simulink model "c00019M_harness"  (R2018a)
settings: Solver=ode3  StartTime=0.0  StopTime=10.0  RelTol=1e-3  EnableMultiTasking=on
undefined symbols (not defined in the file): b, DiscIntNeverNeededParam, J, K, L, PosMinimaW4, R, sigbuilder_block
(part 13 of 43)

== system c00019M_harness/M094/Cyber ==
  note: Sensors
  note: Inputs For Window1
  note: Inputs for Window 2
  note: Inputs for window 3
  note: Inputs for window 4
  note: Users
  note: Users
  note: Sensors
  note: Users
  note: Sensors
  note: Users
  note: Sensors
  note: USERS
      | ---------------------------------
      | 0: None
      | 1: Ventana Arriba
      | 2: Ventana hasta arriba
      | 3: Ventana abajo
      | 4: Ventana hasta abajo
  note: 1: SUBE
      | 0: PARADO
      | -1 BAJA
  note: D = Driver (W1)
      | P1 = Passenger 1 (W2)
      | P2 = Passenger 2 (W3)
      | P3 = Passenger 3 (W4)
      | O = Obstacle
      | C = Control
      | Pri = Prioritizer
      | LD = LockDriver
      | PosW = PositionWindow
      | WL = WindowLogic
      | OW = ObstacleWindow
      | CWXC = ControlWindowXCentralized
      | S = Sensor
      | L = Lock
      | WPos = WindowPosition
      | M = Memory
      | InW = InputWindow
      | WIn = WindowInput
  PosW1 : Inport
  PosW2 : Inport  Port=2
  PosW4 : Inport  Port=3
  DW1 : Inport  Port=4
  P1W2 : Inport  Port=5
  P3W4 : Inport  Port=6
  OW1 : Inport  Port=7
  OW2 : Inport  Port=8
  OW4 : Inport  Port=9
  LD : Inport  Port=10
  CW1C : Inport  Port=11
  CW2C : Inport  Port=12
  CW4C : Inport  Port=13
  Pri : Subsystem
  Pri3 : Subsystem
  Pri4 : Subsystem
  WL : Subsystem
  WL1 : Subsystem
  WL3 : Subsystem
  W1 : Outport
  W2 : Outport  Port=2
  W4 : Outport  Port=3
  wires:
  CW4C/1 -> Pri4/2(CW4C)
  CW2C/1 -> Pri/2(CW2C)
  CW1C/1 -> Pri3/2(CW1C)
  Pri3/1(User) -> WL/2(User)
  WL3/1(WindowLogicOutput) -> W4/1
  Pri4/1(User) -> WL3/2(User)
  OW4/1 -> WL3/3(OW)
  PosW4/1 -> WL3/1(WPos)
  P3W4/1 -> Pri4/1(P)
  WL1/1(WindowLogicOutput) -> W2/1
  OW2/1 -> WL1/3(OW)
  PosW2/1 -> WL1/1(WPos)
  P1W2/1 -> Pri/1(P)
  Pri/1(User) -> WL1/2(User)
  WL/1(WindowLogicOutput) -> W1/1
  DW1/1 -> Pri3/1(D)
  OW1/1 -> WL/3(OW)
  PosW1/1 -> WL/1(WPos)
  LD/1 -> WL3/4(L)

== system c00019M_harness/M094/Physical ==
  InW1 : Inport
  InW2 : Inport  Port=2
  InW4 : Inport  Port=3
  W : Subsystem
  W5 : Subsystem
  W7 : Subsystem
  W1 : Outport
  W2 : Outport  Port=2
  W4 : Outport  Port=3
  wires:
  W7/1(WPos) -> W4/1
  W5/1(WPos) -> W2/1
  W/1(WPos) -> W1/1
  InW4/1 -> W7/1(WIn)
  InW2/1 -> W5/1(WIn)
  InW1/1 -> W/1(WIn)

== system c00019M_harness/M094/S1 ==
  PhyMeasure : Inport
  SensorOut : Outport
  wires:
  PhyMeasure/1 -> SensorOut/1

== system c00019M_harness/M094/S2 ==
  PhyMeasure : Inport
  SensorOut : Outport
  wires:
  PhyMeasure/1 -> SensorOut/1

== system c00019M_harness/M094/S4 ==
  PhyMeasure : Inport
  SensorOut : Outport
  wires:
  PhyMeasure/1 -> SensorOut/1

== system c00019M_harness/M095/Cyber ==
  note: Sensors
  note: Inputs For Window1
  note: Inputs for Window 2
  note: Inputs for window 3
  note: Inputs for window 4
  note: Users
  note: Users
  note: Sensors
  note: Users
  note: Sensors
  note: Users
  note: Sensors
  note: USERS
      | ---------------------------------
      | 0: None
      | 1: Ventana Arriba
      | 2: Ventana hasta arriba
      | 3: Ventana abajo
      | 4: Ventana hasta abajo
  note: 1: SUBE
      | 0: PARADO
      | -1 BAJA
  note: D = Driver (W1)
      | P1 = Passenger 1 (W2)
      | P2 = Passenger 2 (W3)
      | P3 = Passenger 3 (W4)
      | O = Obstacle
      | C = Control
      | Pri = Prioritizer
      | LD = LockDriver
      | PosW = PositionWindow
      | WL = WindowLogic
      | OW = ObstacleWindow
      | CWXC = ControlWindowXCentralized
      | S = Sensor
      | L = Lock
      | WPos = WindowPosition
      | M = Memory
      | InW = InputWindow
      | WIn = WindowInput
  PosW1 : Inport
  PosW2 : Inport  Port=2
  PosW4 : Inport  Port=3
  DW1 : Inport  Port=4
  P1W2 : Inport  Port=5
  P3W4 : Inport  Port=6
  OW1 : Inport  Port=7
  OW2 : Inport  Port=8
  OW4 : Inport  Port=9
  LD : Inport  Port=10
  CW1C : Inport  Port=11
  CW2C : Inport  Port=12
  CW4C : Inport  Port=13
  Pri : Subsystem
  Pri3 : Subsystem
  Pri4 : Subsystem
  WL : Subsystem
  WL1 : Subsystem
  WL3 : Subsystem
  W1 : Outport
  W2 : Outport  Port=2
  W4 : Outport  Port=3
  wires:
  CW4C/1 -> Pri4/2(CW4C)
  CW2C/1 -> Pri/2(CW2C)
  CW1C/1 -> Pri3/2(CW1C)
  Pri3/1(User) -> WL/2(User)
  WL3/1(WindowLogicOutput) -> W4/1
  Pri4/1(User) -> WL3/2(User)
  OW4/1 -> WL3/3(OW)
  PosW4/1 -> WL3/1(WPos)
  P3W4/1 -> Pri4/1(P)
  WL1/1(WindowLogicOutput) -> W2/1
  OW2/1 -> WL1/3(OW)
  PosW2/1 -> WL1/1(WPos)
  P1W2/1 -> Pri/1(P)
  Pri/1(User) -> WL1/2(User)
  WL/1(WindowLogicOutput) -> W1/1
  DW1/1 -> Pri3/1(D)
  OW1/1 -> WL/3(OW)
  PosW1/1 -> WL/1(WPos)
  LD/1 -> WL3/4(L)

== system c00019M_harness/M095/Physical ==
  InW1 : Inport
  InW2 : Inport  Port=2
  InW4 : Inport  Port=3
  W : Subsystem
  W5 : Subsystem
  W7 : Subsystem
  W1 : Outport
  W2 : Outport  Port=2
  W4 : Outport  Port=3
  wires:
  W7/1(WPos) -> W4/1
  W5/1(WPos) -> W2/1
  W/1(WPos) -> W1/1
  InW4/1 -> W7/1(WIn)
  InW2/1 -> W5/1(WIn)
  InW1/1 -> W/1(WIn)

== system c00019M_harness/M095/S1 ==
  PhyMeasure : Inport
  SensorOut : Outport
  wires:
  PhyMeasure/1 -> SensorOut/1

== system c00019M_harness/M095/S2 ==
  PhyMeasure : Inport
  SensorOut : Outport
  wires:
  PhyMeasure/1 -> SensorOut/1

== system c00019M_harness/M095/S4 ==
  PhyMeasure : Inport
  SensorOut : Outport
  wires:
  PhyMeasure/1 -> SensorOut/1

== system c00019M_harness/M096/Cyber ==
  note: Sensors
  note: Inputs For Window1
  note: Inputs for Window 2
  note: Inputs for window 3
  note: Inputs for window 4
  note: Users
  note: Users
  note: Sensors
  note: Users
  note: Sensors
  note: Users
  note: Sensors
  note: USERS
      | ---------------------------------
      | 0: None
      | 1: Ventana Arriba
      | 2: Ventana hasta arriba
      | 3: Ventana abajo
      | 4: Ventana hasta abajo
  note: 1: SUBE
      | 0: PARADO
      | -1 BAJA
  note: D = Driver (W1)
      | P1 = Passenger 1 (W2)
      | P2 = Passenger 2 (W3)
      | P3 = Passenger 3 (W4)
      | O = Obstacle
      | C = Control
      | Pri = Prioritizer
      | LD = LockDriver
      | PosW = PositionWindow
      | WL = WindowLogic
      | OW = ObstacleWindow
      | CWXC = ControlWindowXCentralized
      | S = Sensor
      | L = Lock
      | WPos = WindowPosition
      | M = Memory
      | InW = InputWindow
      | WIn = WindowInput
  PosW1 : Inport
  PosW2 : Inport  Port=2
  PosW4 : Inport  Port=3
  DW1 : Inport  Port=4
  P1W2 : Inport  Port=5
  P3W4 : Inport  Port=6
  OW1 : Inport  Port=7
  OW2 : Inport  Port=8
  OW4 : Inport  Port=9
  LD : Inport  Port=10
  CW1C : Inport  Port=11
  CW2C : Inport  Port=12
  CW4C : Inport  Port=13
  Pri : Subsystem
  Pri3 : Subsystem
  Pri4 : Subsystem
  WL : Subsystem
  WL1 : Subsystem
  WL3 : Subsystem
  W1 : Outport
  W2 : Outport  Port=2
  W4 : Outport  Port=3
  wires:
  CW4C/1 -> Pri4/2(CW4C)
  CW2C/1 -> Pri/2(CW2C)
  CW1C/1 -> Pri3/2(CW1C)
  Pri3/1(User) -> WL/2(User)
  WL3/1(WindowLogicOutput) -> W4/1
  Pri4/1(User) -> WL3/2(User)
  OW4/1 -> WL3/3(OW)
  PosW4/1 -> WL3/1(WPos)
  P3W4/1 -> Pri4/1(P)
  WL1/1(WindowLogicOutput) -> W2/1
  OW2/1 -> WL1/3(OW)
  PosW2/1 -> WL1/1(WPos)
  P1W2/1 -> Pri/1(P)
  Pri/1(User) -> WL1/2(User)
  WL/1(WindowLogicOutput) -> W1/1
  DW1/1 -> Pri3/1(D)
  OW1/1 -> WL/3(OW)
  PosW1/1 -> WL/1(WPos)
  LD/1 -> WL3/4(L)

== system c00019M_harness/M096/Physical ==
  InW1 : Inport
  InW2 : Inport  Port=2
  InW4 : Inport  Port=3
  W : Subsystem
  W5 : Subsystem
  W7 : Subsystem
  W1 : Outport
  W2 : Outport  Port=2
  W4 : Outport  Port=3
  wires:
  W7/1(WPos) -> W4/1
  W5/1(WPos) -> W2/1
  W/1(WPos) -> W1/1
  InW4/1 -> W7/1(WIn)
  InW2/1 -> W5/1(WIn)
  InW1/1 -> W/1(WIn)

== system c00019M_harness/M096/S1 ==
  PhyMeasure : Inport
  SensorOut : Outport
  wires:
  PhyMeasure/1 -> SensorOut/1

== system c00019M_harness/M096/S2 ==
  PhyMeasure : Inport
  SensorOut : Outport
  wires:
  PhyMeasure/1 -> SensorOut/1

== system c00019M_harness/M096/S4 ==
  PhyMeasure : Inport
  SensorOut : Outport
  wires:
  PhyMeasure/1 -> SensorOut/1

== system c00019M_harness/M098/Cyber ==
  note: Sensors
  note: Inputs For Window1
  note: Inputs for Window 2
  note: Inputs for window 3
  note: Inputs for window 4
  note: Users
  note: Users
  note: Sensors
  note: Users
  note: Sensors
  note: Users
  note: Sensors
  note: USERS
      | ---------------------------------
      | 0: None
      | 1: Ventana Arriba
      | 2: Ventana hasta arriba
      | 3: Ventana abajo
      | 4: Ventana hasta abajo
  note: 1: SUBE
      | 0: PARADO
      | -1 BAJA
  note: D = Driver (W1)
      | P1 = Passenger 1 (W2)
      | P2 = Passenger 2 (W3)
      | P3 = Passenger 3 (W4)
      | O = Obstacle
      | C = Control
      | Pri = Prioritizer
      | LD = LockDriver
      | PosW = PositionWindow
      | WL = WindowLogic
      | OW = ObstacleWindow
      | CWXC = ControlWindowXCentralized
      | S = Sensor
      | L = Lock
      | WPos = WindowPosition
      | M = Memory
      | InW = InputWindow
      | WIn = WindowInput
  PosW1 : Inport
  PosW2 : Inport  Port=2
  PosW4 : Inport  Port=3
  DW1 : Inport  Port=4
  P1W2 : Inport  Port=5
  P3W4 : Inport  Port=6
  OW1 : Inport  Port=7
  OW2 : Inport  Port=8
  OW4 : Inport  Port=9
  LD : Inport  Port=10
  CW1C : Inport  Port=11
  CW2C : Inport  Port=12
  CW4C : Inport  Port=13
  Pri : Subsystem
  Pri3 : Subsystem
  Pri4 : Subsystem
  WL : Subsystem
  WL1 : Subsystem
  WL3 : Subsystem
  W1 : Outport
  W2 : Outport  Port=2
  W4 : Outport  Port=3
  wires:
  CW4C/1 -> Pri4/2(CW4C)
  CW2C/1 -> Pri/2(CW2C)
  CW1C/1 -> Pri3/2(CW1C)
  Pri3/1(User) -> WL/2(User)
  WL3/1(WindowLogicOutput) -> W4/1
  Pri4/1(User) -> WL3/2(User)
  OW4/1 -> WL3/3(OW)
  PosW4/1 -> WL3/1(WPos)
  P3W4/1 -> Pri4/1(P)
  WL1/1(WindowLogicOutput) -> W2/1
  OW2/1 -> WL1/3(OW)
  PosW2/1 -> WL1/1(WPos)
  P1W2/1 -> Pri/1(P)
  Pri/1(User) -> WL1/2(User)
  WL/1(WindowLogicOutput) -> W1/1
  DW1/1 -> Pri3/1(D)
  OW1/1 -> WL/3(OW)
  PosW1/1 -> WL/1(WPos)
  LD/1 -> WL3/4(L)

== system c00019M_harness/M098/Physical ==
  InW1 : Inport
  InW2 : Inport  Port=2
  InW4 : Inport  Port=3
  W : Subsystem
  W5 : Subsystem
  W7 : Subsystem
  W1 : Outport
  W2 : Outport  Port=2
  W4 : Outport  Port=3
  wires:
  W7/1(WPos) -> W4/1
  W5/1(WPos) -> W2/1
  W/1(WPos) -> W1/1
  InW4/1 -> W7/1(WIn)
  InW2/1 -> W5/1(WIn)
  InW1/1 -> W/1(WIn)

== system c00019M_harness/M098/S1 ==
  PhyMeasure : Inport
  SensorOut : Outport
  wires:
  PhyMeasure/1 -> SensorOut/1

== system c00019M_harness/M098/S2 ==
  PhyMeasure : Inport
  SensorOut : Outport
  wires:
  PhyMeasure/1 -> SensorOut/1

== system c00019M_harness/M098/S4 ==
  PhyMeasure : Inport
  SensorOut : Outport
  wires:
  PhyMeasure/1 -> SensorOut/1

== system c00019M_harness/M099/Cyber ==
  note: Sensors
  note: Inputs For Window1
  note: Inputs for Window 2
  note: Inputs for window 3
  note: Inputs for window 4
  note: Users
  note: Users
  note: Sensors
  note: Users
  note: Sensors
  note: Users
  note: Sensors
  note: USERS
      | ---------------------------------
      | 0: None
      | 1: Ventana Arriba
      | 2: Ventana hasta arriba
      | 3: Ventana abajo
      | 4: Ventana hasta abajo
  note: 1: SUBE
      | 0: PARADO
      | -1 BAJA
  note: D = Driver (W1)
      | P1 = Passenger 1 (W2)
      | P2 = Passenger 2 (W3)
      | P3 = Passenger 3 (W4)
      | O = Obstacle
      | C = Control
      | Pri = Prioritizer
      | LD = LockDriver
      | PosW = PositionWindow
      | WL = WindowLogic
      | OW = ObstacleWindow
      | CWXC = ControlWindowXCentralized
      | S = Sensor
      | L = Lock
      | WPos = WindowPosition
      | M = Memory
      | InW = InputWindow
      | WIn = WindowInput
  PosW1 : Inport
  PosW2 : Inport  Port=2
  PosW4 : Inport  Port=3
  DW1 : Inport  Port=4
  P1W2 : Inport  Port=5
  P3W4 : Inport  Port=6
  OW1 : Inport  Port=7
  OW2 : Inport  Port=8
  OW4 : Inport  Port=9
  LD : Inport  Port=10
  CW1C : Inport  Port=11
  CW2C : Inport  Port=12
  CW4C : Inport  Port=13
  Pri : Subsystem
  Pri3 : Subsystem
  Pri4 : Subsystem
  WL : Subsystem
  WL1 : Subsystem
  WL3 : Subsystem
  W1 : Outport
  W2 : Outport  Port=2
  W4 : Outport  Port=3
  wires:
  CW4C/1 -> Pri4/2(CW4C)
  CW2C/1 -> Pri/2(CW2C)
  CW1C/1 -> Pri3/2(CW1C)
  Pri3/1(User) -> WL/2(User)
  WL3/1(WindowLogicOutput) -> W4/1
  Pri4/1(User) -> WL3/2(User)
  OW4/1 -> WL3/3(OW)
  PosW4/1 -> WL3/1(WPos)
  P3W4/1 -> Pri4/1(P)
  WL1/1(WindowLogicOutput) -> W2/1
  OW2/1 -> WL1/3(OW)
  PosW2/1 -> WL1/1(WPos)
  P1W2/1 -> Pri/1(P)
  Pri/1(User) -> WL1/2(User)
  WL/1(WindowLogicOutput) -> W1/1
  DW1/1 -> Pri3/1(D)
  OW1/1 -> WL/3(OW)
  PosW1/1 -> WL/1(WPos)
  LD/1 -> WL3/4(L)

== system c00019M_harness/M099/Physical ==
  InW1 : Inport
  InW2 : Inport  Port=2
  InW4 : Inport  Port=3
  W : Subsystem
  W5 : Subsystem
  W7 : Subsystem
  W1 : Outport
  W2 : Outport  Port=2
  W4 : Outport  Port=3
  wires:
  W7/1(WPos) -> W4/1
  W5/1(WPos) -> W2/1
  W/1(WPos) -> W1/1
  InW4/1 -> W7/1(WIn)
  InW2/1 -> W5/1(WIn)
  InW1/1 -> W/1(WIn)

== system c00019M_harness/M099/S1 ==
  PhyMeasure : Inport
  SensorOut : Outport
  wires:
  PhyMeasure/1 -> SensorOut/1

== system c00019M_harness/M099/S2 ==
  PhyMeasure : Inport
  SensorOut : Outport
  wires:
  PhyMeasure/1 -> SensorOut/1

== system c00019M_harness/M099/S4 ==
  PhyMeasure : Inport
  SensorOut : Outport
  wires:
  PhyMeasure/1 -> SensorOut/1

== system c00019M_harness/M100/Cyber ==
  note: Sensors
  note: Inputs For Window1
  note: Inputs for Window 2
  note: Inputs for window 3
  note: Inputs for window 4
  note: Users
  note: Users
  note: Sensors
  note: Users
  note: Sensors
  note: Users
  note: Sensors
  note: USERS
      | ---------------------------------
      | 0: None
      | 1: Ventana Arriba
      | 2: Ventana hasta arriba
      | 3: Ventana abajo
      | 4: Ventana hasta abajo
  note: 1: SUBE
      | 0: PARADO
      | -1 BAJA
  note: D = Driver (W1)
      | P1 = Passenger 1 (W2)
      | P2 = Passenger 2 (W3)
      | P3 = Passenger 3 (W4)
      | O = Obstacle
      | C = Control
      | Pri = Prioritizer
      | LD = LockDriver
      | PosW = PositionWindow
      | WL = WindowLogic
      | OW = ObstacleWindow
      | CWXC = ControlWindowXCentralized
      | S = Sensor
      | L = Lock
      | WPos = WindowPosition
      | M = Memory
      | InW = InputWindow
      | WIn = WindowInput
  PosW1 : Inport
  PosW2 : Inport  Port=2
  PosW4 : Inport  Port=3
  DW1 : Inport  Port=4
  P1W2 : Inport  Port=5
  P3W4 : Inport  Port=6
  OW1 : Inport  Port=7
  OW2 : Inport  Port=8
  OW4 : Inport  Port=9
  LD : Inport  Port=10
  CW1C : Inport  Port=11
  CW2C : Inport  Port=12
  CW4C : Inport  Port=13
  Pri : Subsystem
  Pri3 : Subsystem
  Pri4 : Subsystem
  WL : Subsystem
  WL1 : Subsystem
  WL3 : Subsystem
  W1 : Outport
  W2 : Outport  Port=2
  W4 : Outport  Port=3
  wires:
  CW4C/1 -> Pri4/2(CW4C)
  CW2C/1 -> Pri/2(CW2C)
  CW1C/1 -> Pri3/2(CW1C)
  Pri3/1(User) -> WL/2(User)
  WL3/1(WindowLogicOutput) -> W4/1
  Pri4/1(User) -> WL3/2(User)
  OW4/1 -> WL3/3(OW)
  PosW4/1 -> WL3/1(WPos)
  P3W4/1 -> Pri4/1(P)
  WL1/1(WindowLogicOutput) -> W2/1
  OW2/1 -> WL1/3(OW)
  PosW2/1 -> WL1/1(WPos)
  P1W2/1 -> Pri/1(P)
  Pri/1(User) -> WL1/2(User)
  WL/1(WindowLogicOutput) -> W1/1
  DW1/1 -> Pri3/1(D)
  OW1/1 -> WL/3(OW)
  PosW1/1 -> WL/1(WPos)
  LD/1 -> WL3/4(L)

== system c00019M_harness/M100/Physical ==
  InW1 : Inport
  InW2 : Inport  Port=2
  InW4 : Inport  Port=3
  W : Subsystem
  W5 : Subsystem
  W7 : Subsystem
  W1 : Outport
  W2 : Outport  Port=2
  W4 : Outport  Port=3
  wires:
  W7/1(WPos) -> W4/1
  W5/1(WPos) -> W2/1
  W/1(WPos) -> W1/1
  InW4/1 -> W7/1(WIn)
  InW2/1 -> W5/1(WIn)
  InW1/1 -> W/1(WIn)

== system c00019M_harness/M100/S1 ==
  PhyMeasure : Inport
  SensorOut : Outport
  wires:
  PhyMeasure/1 -> SensorOut/1

== system c00019M_harness/M100/S2 ==
  PhyMeasure : Inport
  SensorOut : Outport
  wires:
  PhyMeasure/1 -> SensorOut/1

== system c00019M_harness/M100/S4 ==
  PhyMeasure : Inport
  SensorOut : Outport
  wires:
  PhyMeasure/1 -> SensorOut/1

== system c00019M_harness/M102/Cyber ==
  note: Sensors
  note: Inputs For Window1
  note: Inputs for Window 2
  note: Inputs for window 3
  note: Inputs for window 4
  note: Users
  note: Users
  note: Sensors
  note: Users
  note: Sensors
  note: Users
  note: Sensors
  note: USERS
      | ---------------------------------
      | 0: None
      | 1: Ventana Arriba
      | 2: Ventana hasta arriba
      | 3: Ventana abajo
      | 4: Ventana hasta abajo
  note: 1: SUBE
      | 0: PARADO
      | -1 BAJA
  note: D = Driver (W1)
      | P1 = Passenger 1 (W2)
      | P2 = Passenger 2 (W3)
      | P3 = Passenger 3 (W4)
      | O = Obstacle
      | C = Control
      | Pri = Prioritizer
      | LD = LockDriver
      | PosW = PositionWindow
      | WL = WindowLogic
      | OW = ObstacleWindow
      | CWXC = ControlWindowXCentralized
      | S = Sensor
      | L = Lock
      | WPos = WindowPosition
      | M = Memory
      | InW = InputWindow
      | WIn = WindowInput
  PosW1 : Inport
  PosW2 : Inport  Port=2
  PosW4 : Inport  Port=3
  DW1 : Inport  Port=4
  P1W2 : Inport  Port=5
  P3W4 : Inport  Port=6
  OW1 : Inport  Port=7
  OW2 : Inport  Port=8
  OW4 : Inport  Port=9
  LD : Inport  Port=10
  CW1C : Inport  Port=11
  CW2C : Inport  Port=12
  CW4C : Inport  Port=13
  Pri : Subsystem
  Pri3 : Subsystem
  Pri4 : Subsystem
  WL : Subsystem
  WL1 : Subsystem
  WL3 : Subsystem
  W1 : Outport
  W2 : Outport  Port=2
  W4 : Outport  Port=3
  wires:
  CW4C/1 -> Pri4/2(CW4C)
  CW2C/1 -> Pri/2(CW2C)
  CW1C/1 -> Pri3/2(CW1C)
  Pri3/1(User) -> WL/2(User)
  WL3/1(WindowLogicOutput) -> W4/1
  Pri4/1(User) -> WL3/2(User)
  OW4/1 -> WL3/3(OW)
  PosW4/1 -> WL3/1(WPos)
  P3W4/1 -> Pri4/1(P)
  WL1/1(WindowLogicOutput) -> W2/1
  OW2/1 -> WL1/3(OW)
  PosW2/1 -> WL1/1(WPos)
  P1W2/1 -> Pri/1(P)
  Pri/1(User) -> WL1/2(User)
  WL/1(WindowLogicOutput) -> W1/1
  DW1/1 -> Pri3/1(D)
  OW1/1 -> WL/3(OW)
  PosW1/1 -> WL/1(WPos)
  LD/1 -> WL3/4(L)

== system c00019M_harness/M102/Physical ==
  InW1 : Inport
  InW2 : Inport  Port=2
  InW4 : Inport  Port=3
  W : Subsystem
  W5 : Subsystem
  W7 : Subsystem
  W1 : Outport
  W2 : Outport  Port=2
  W4 : Outport  Port=3
  wires:
  W7/1(WPos) -> W4/1
  W5/1(WPos) -> W2/1
  W/1(WPos) -> W1/1
  InW4/1 -> W7/1(WIn)
  InW2/1 -> W5/1(WIn)
  InW1/1 -> W/1(WIn)

== system c00019M_harness/M102/S1 ==
  PhyMeasure : Inport
  SensorOut : Outport
  wires:
  PhyMeasure/1 -> SensorOut/1

== system c00019M_harness/M102/S2 ==
  PhyMeasure : Inport
  SensorOut : Outport
  wires:
  PhyMeasure/1 -> SensorOut/1

== system c00019M_harness/M102/S4 ==
  PhyMeasure : Inport
  SensorOut : Outport
  wires:
  PhyMeasure/1 -> SensorOut/1

== system c00019M_harness/M103/Cyber ==
  note: Sensors
  note: Inputs For Window1
  note: Inputs for Window 2
  note: Inputs for window 3
  note: Inputs for window 4
  note: Users
  note: Users
  note: Sensors
  note: Users
  note: Sensors
  note: Users
  note: Sensors
  note: USERS
      | ---------------------------------
      | 0: None
      | 1: Ventana Arriba
      | 2: Ventana hasta arriba
      | 3: Ventana abajo
      | 4: Ventana hasta abajo
  note: 1: SUBE
      | 0: PARADO
      | -1 BAJA
  note: D = Driver (W1)
      | P1 = Passenger 1 (W2)
      | P2 = Passenger 2 (W3)
      | P3 = Passenger 3 (W4)
      | O = Obstacle
      | C = Control
      | Pri = Prioritizer
      | LD = LockDriver
      | PosW = PositionWindow
      | WL = WindowLogic
      | OW = ObstacleWindow
      | CWXC = ControlWindowXCentralized
      | S = Sensor
      | L = Lock
      | WPos = WindowPosition
      | M = Memory
      | InW = InputWindow
      | WIn = WindowInput
  PosW1 : Inport
  PosW2 : Inport  Port=2
  PosW4 : Inport  Port=3
  DW1 : Inport  Port=4
  P1W2 : Inport  Port=5
  P3W4 : Inport  Port=6
  OW1 : Inport  Port=7
  OW2 : Inport  Port=8
  OW4 : Inport  Port=9
  LD : Inport  Port=10
  CW1C : Inport  Port=11
  CW2C : Inport  Port=12
  CW4C : Inport  Port=13
  Pri : Subsystem
  Pri3 : Subsystem
  Pri4 : Subsystem
  WL : Subsystem
  WL1 : Subsystem
  WL3 : Subsystem
  W1 : Outport
  W2 : Outport  Port=2
  W4 : Outport  Port=3
  wires:
  CW4C/1 -> Pri4/2(CW4C)
  CW2C/1 -> Pri/2(CW2C)
  CW1C/1 -> Pri3/2(CW1C)
  Pri3/1(User) -> WL/2(User)
  WL3/1(WindowLogicOutput) -> W4/1
  Pri4/1(User) -> WL3/2(User)
  OW4/1 -> WL3/3(OW)
  PosW4/1 -> WL3/1(WPos)
  P3W4/1 -> Pri4/1(P)
  WL1/1(WindowLogicOutput) -> W2/1
  OW2/1 -> WL1/3(OW)
  PosW2/1 -> WL1/1(WPos)
  P1W2/1 -> Pri/1(P)
  Pri/1(User) -> WL1/2(User)
  WL/1(WindowLogicOutput) -> W1/1
  DW1/1 -> Pri3/1(D)
  OW1/1 -> WL/3(OW)
  PosW1/1 -> WL/1(WPos)
  LD/1 -> WL3/4(L)

== system c00019M_harness/M103/Physical ==
  InW1 : Inport
  InW2 : Inport  Port=2
  InW4 : Inport  Port=3
  W : Subsystem
  W5 : Subsystem
  W7 : Subsystem
  W1 : Outport
  W2 : Outport  Port=2
  W4 : Outport  Port=3
  wires:
  W7/1(WPos) -> W4/1
  W5/1(WPos) -> W2/1
  W/1(WPos) -> W1/1
  InW4/1 -> W7/1(WIn)
  InW2/1 -> W5/1(WIn)
  InW1/1 -> W/1(WIn)

== system c00019M_harness/M103/S1 ==
  PhyMeasure : Inport
  SensorOut : Outport
  wires:
  PhyMeasure/1 -> SensorOut/1

== system c00019M_harness/M103/S2 ==
  PhyMeasure : Inport
  SensorOut : Outport
  wires:
  PhyMeasure/1 -> SensorOut/1

== system c00019M_harness/M103/S4 ==
  PhyMeasure : Inport
  SensorOut : Outport
  wires:
  PhyMeasure/1 -> SensorOut/1

== system c00019M_harness/M104/Cyber ==
  note: Sensors
  note: Inputs For Window1
  note: Inputs for Window 2
  note: Inputs for window 3
  note: Inputs for window 4
  note: Users
  note: Users
  note: Sensors
  note: Users
  note: Sensors
  note: Users
  note: Sensors
  note: USERS
      | ---------------------------------
      | 0: None
      | 1: Ventana Arriba
      | 2: Ventana hasta arriba
      | 3: Ventana abajo
      | 4: Ventana hasta abajo
  note: 1: SUBE
      | 0: PARADO
      | -1 BAJA
  note: D = Driver (W1)
      | P1 = Passenger 1 (W2)
      | P2 = Passenger 2 (W3)
      | P3 = Passenger 3 (W4)
      | O = Obstacle
      | C = Control
      | Pri = Prioritizer
      | LD = LockDriver
      | PosW = PositionWindow
      | WL = WindowLogic
      | OW = ObstacleWindow
      | CWXC = ControlWindowXCentralized
      | S = Sensor
      | L = Lock
      | WPos = WindowPosition
      | M = Memory
      | InW = InputWindow
      | WIn = WindowInput
  PosW1 : Inport
  PosW2 : Inport  Port=2
  PosW4 : Inport  Port=3
  DW1 : Inport  Port=4
  P1W2 : Inport  Port=5
  P3W4 : Inport  Port=6
  OW1 : Inport  Port=7
  OW2 : Inport  Port=8
  OW4 : Inport  Port=9
  LD : Inport  Port=10
  CW1C : Inport  Port=11
  CW2C : Inport  Port=12
  CW4C : Inport  Port=13
  Pri : Subsystem
  Pri3 : Subsystem
  Pri4 : Subsystem
  WL : Subsystem
  WL1 : Subsystem
  WL3 : Subsystem
  W1 : Outport
  W2 : Outport  Port=2
  W4 : Outport  Port=3
  wires:
  CW4C/1 -> Pri4/2(CW4C)
  CW2C/1 -> Pri/2(CW2C)
  CW1C/1 -> Pri3/2(CW1C)
  Pri3/1(User) -> WL/2(User)
  WL3/1(WindowLogicOutput) -> W4/1
  Pri4/1(User) -> WL3/2(User)
  OW4/1 -> WL3/3(OW)
  PosW4/1 -> WL3/1(WPos)
  P3W4/1 -> Pri4/1(P)
  WL1/1(WindowLogicOutput) -> W2/1
  OW2/1 -> WL1/3(OW)
  PosW2/1 -> WL1/1(WPos)
  P1W2/1 -> Pri/1(P)
  Pri/1(User) -> WL1/2(User)
  WL/1(WindowLogicOutput) -> W1/1
  DW1/1 -> Pri3/1(D)
  OW1/1 -> WL/3(OW)
  PosW1/1 -> WL/1(WPos)
  LD/1 -> WL3/4(L)

== system c00019M_harness/M104/Physical ==
  InW1 : Inport
  InW2 : Inport  Port=2
  InW4 : Inport  Port=3
  W : Subsystem
  W5 : Subsystem
  W7 : Subsystem
  W1 : Outport
  W2 : Outport  Port=2
  W4 : Outport  Port=3
  wires:
  W7/1(WPos) -> W4/1
  W5/1(WPos) -> W2/1
  W/1(WPos) -> W1/1
  InW4/1 -> W7/1(WIn)
  InW2/1 -> W5/1(WIn)
  InW1/1 -> W/1(WIn)

== system c00019M_harness/M104/S1 ==
  PhyMeasure : Inport
  SensorOut : Outport
  wires:
  PhyMeasure/1 -> SensorOut/1

== system c00019M_harness/M104/S2 ==
  PhyMeasure : Inport
  SensorOut : Outport
  wires:
  PhyMeasure/1 -> SensorOut/1

== system c00019M_harness/M104/S4 ==
  PhyMeasure : Inport
  SensorOut : Outport
  wires:
  PhyMeasure/1 -> SensorOut/1

== system c00019M_harness/M106/Cyber ==
  note: Sensors
  note: Inputs For Window1
  note: Inputs for Window 2
  note: Inputs for window 3
  note: Inputs for window 4
  note: Users
  note: Users
  note: Sensors
  note: Users
  note: Sensors
  note: Users
  note: Sensors
  note: USERS
      | ---------------------------------
      | 0: None
      | 1: Ventana Arriba
      | 2: Ventana hasta arriba
      | 3: Ventana abajo
      | 4: Ventana hasta abajo
  note: 1: SUBE
      | 0: PARADO
      | -1 BAJA
  note: D = Driver (W1)
      | P1 = Passenger 1 (W2)
      | P2 = Passenger 2 (W3)
      | P3 = Passenger 3 (W4)
      | O = Obstacle
      | C = Control
      | Pri = Prioritizer
      | LD = LockDriver
      | PosW = PositionWindow
      | WL = WindowLogic
      | OW = ObstacleWindow
      | CWXC = ControlWindowXCentralized
      | S = Sensor
      | L = Lock
      | WPos = WindowPosition
      | M = Memory
      | InW = InputWindow
      | WIn = WindowInput
  PosW1 : Inport
  PosW2 : Inport  Port=2
  PosW4 : Inport  Port=3
  DW1 : Inport  Port=4
  P1W2 : Inport  Port=5
  P3W4 : Inport  Port=6
  OW1 : Inport  Port=7
  OW2 : Inport  Port=8
  OW4 : Inport  Port=9
  LD : Inport  Port=10
  CW1C : Inport  Port=11
  CW2C : Inport  Port=12
  CW4C : Inport  Port=13
  Pri : Subsystem
  Pri3 : Subsystem
  Pri4 : Subsystem
  WL : Subsystem
  WL1 : Subsystem
  WL3 : Subsystem
  W1 : Outport
  W2 : Outport  Port=2
  W4 : Outport  Port=3
  wires:
  CW4C/1 -> Pri4/2(CW4C)
  CW2C/1 -> Pri/2(CW2C)
  CW1C/1 -> Pri3/2(CW1C)
  Pri3/1(User) -> WL/2(User)
  WL3/1(WindowLogicOutput) -> W4/1
  Pri4/1(User) -> WL3/2(User)
  OW4/1 -> WL3/3(OW)
  PosW4/1 -> WL3/1(WPos)
  P3W4/1 -> Pri4/1(P)
  WL1/1(WindowLogicOutput) -> W2/1
  OW2/1 -> WL1/3(OW)
  PosW2/1 -> WL1/1(WPos)
  P1W2/1 -> Pri/1(P)
  Pri/1(User) -> WL1/2(User)
  WL/1(WindowLogicOutput) -> W1/1
  DW1/1 -> Pri3/1(D)
  OW1/1 -> WL/3(OW)
  PosW1/1 -> WL/1(WPos)
  LD/1 -> WL3/4(L)

== system c00019M_harness/M106/Physical ==
  InW1 : Inport
  InW2 : Inport  Port=2
  InW4 : Inport  Port=3
  W : Subsystem
  W5 : Subsystem
  W7 : Subsystem
  W1 : Outport
  W2 : Outport  Port=2
  W4 : Outport  Port=3
  wires:
  W7/1(WPos) -> W4/1
  W5/1(WPos) -> W2/1
  W/1(WPos) -> W1/1
  InW4/1 -> W7/1(WIn)
  InW2/1 -> W5/1(WIn)
  InW1/1 -> W/1(WIn)

== system c00019M_harness/M106/S1 ==
  PhyMeasure : Inport
  SensorOut : Outport
  wires:
  PhyMeasure/1 -> SensorOut/1

== system c00019M_harness/M106/S2 ==
  PhyMeasure : Inport
  SensorOut : Outport
  wires:
  PhyMeasure/1 -> SensorOut/1

== system c00019M_harness/M106/S4 ==
  PhyMeasure : Inport
  SensorOut : Outport
  wires:
  PhyMeasure/1 -> SensorOut/1

== system c00019M_harness/M107/Cyber ==
  note: Sensors
  note: Inputs For Window1
  note: Inputs for Window 2
  note: Inputs for window 3
  note: Inputs for window 4
  note: Users
  note: Users
  note: Sensors
  note: Users
  note: Sensors
  note: Users
  note: Sensors
  note: USERS
      | ---------------------------------
      | 0: None
      | 1: Ventana Arriba
      | 2: Ventana hasta arriba
      | 3: Ventana abajo
      | 4: Ventana hasta abajo
  note: 1: SUBE
      | 0: PARADO
      | -1 BAJA
  note: D = Driver (W1)
      | P1 = Passenger 1 (W2)
      | P2 = Passenger 2 (W3)
      | P3 = Passenger 3 (W4)
      | O = Obstacle
      | C = Control
      | Pri = Prioritizer
      | LD = LockDriver
      | PosW = PositionWindow
      | WL = WindowLogic
      | OW = ObstacleWindow
      | CWXC = ControlWindowXCentralized
      | S = Sensor
      | L = Lock
      | WPos = WindowPosition
      | M = Memory
      | InW = InputWindow
      | WIn = WindowInput
  PosW1 : Inport
  PosW2 : Inport  Port=2
  PosW4 : Inport  Port=3
  DW1 : Inport  Port=4
  P1W2 : Inport  Port=5
  P3W4 : Inport  Port=6
  OW1 : Inport  Port=7
  OW2 : Inport  Port=8
  OW4 : Inport  Port=9
  LD : Inport  Port=10
  CW1C : Inport  Port=11
  CW2C : Inport  Port=12
  CW4C : Inport  Port=13
  Pri : Subsystem
  Pri3 : Subsystem
  Pri4 : Subsystem
  WL : Subsystem
  WL1 : Subsystem
  WL3 : Subsystem
  W1 : Outport
  W2 : Outport  Port=2
  W4 : Outport  Port=3
  wires:
  CW4C/1 -> Pri4/2(CW4C)
  CW2C/1 -> Pri/2(CW2C)
  CW1C/1 -> Pri3/2(CW1C)
  Pri3/1(User) -> WL/2(User)
  WL3/1(WindowLogicOutput) -> W4/1
  Pri4/1(User) -> WL3/2(User)
  OW4/1 -> WL3/3(OW)
  PosW4/1 -> WL3/1(WPos)
  P3W4/1 -> Pri4/1(P)
  WL1/1(WindowLogicOutput) -> W2/1
  OW2/1 -> WL1/3(OW)
  PosW2/1 -> WL1/1(WPos)
  P1W2/1 -> Pri/1(P)
  Pri/1(User) -> WL1/2(User)
  WL/1(WindowLogicOutput) -> W1/1
  DW1/1 -> Pri3/1(D)
  OW1/1 -> WL/3(OW)
  PosW1/1 -> WL/1(WPos)
  LD/1 -> WL3/4(L)

== system c00019M_harness/M107/Physical ==
  InW1 : Inport
  InW2 : Inport  Port=2
  InW4 : Inport  Port=3
  W : Subsystem
  W5 : Subsystem
  W7 : Subsystem
  W1 : Outport
  W2 : Outport  Port=2
  W4 : Outport  Port=3
  wires:
  W7/1(WPos) -> W4/1
  W5/1(WPos) -> W2/1
  W/1(WPos) -> W1/1
  InW4/1 -> W7/1(WIn)
  InW2/1 -> W5/1(WIn)
  InW1/1 -> W/1(WIn)

== system c00019M_harness/M107/S1 ==
  PhyMeasure : Inport
  SensorOut : Outport
  wires:
  PhyMeasure/1 -> SensorOut/1

== system c00019M_harness/M107/S2 ==
  PhyMeasure : Inport
  SensorOut : Outport
  wires:
  PhyMeasure/1 -> SensorOut/1

== system c00019M_harness/M107/S4 ==
  PhyMeasure : Inport
  SensorOut : Outport
  wires:
  PhyMeasure/1 -> SensorOut/1

== system c00019M_harness/M108/Cyber ==
  note: Sensors
  note: Inputs For Window1
  note: Inputs for Window 2
  note: Inputs for window 3
  note: Inputs for window 4
  note: Users
  note: Users
  note: Sensors
  note: Users
  note: Sensors
  note: Users
  note: Sensors
  note: USERS
      | ---------------------------------
      | 0: None
      | 1: Ventana Arriba
      | 2: Ventana hasta arriba
      | 3: Ventana abajo
      | 4: Ventana hasta abajo
  note: 1: SUBE
      | 0: PARADO
      | -1 BAJA
  note: D = Driver (W1)
      | P1 = Passenger 1 (W2)
      | P2 = Passenger 2 (W3)
      | P3 = Passenger 3 (W4)
      | O = Obstacle
      | C = Control
      | Pri = Prioritizer
      | LD = LockDriver
      | PosW = PositionWindow
      | WL = WindowLogic
      | OW = ObstacleWindow
      | CWXC = ControlWindowXCentralized
      | S = Sensor
      | L = Lock
      | WPos = WindowPosition
      | M = Memory
      | InW = InputWindow
      | WIn = WindowInput
  PosW1 : Inport
  PosW2 : Inport  Port=2
  PosW4 : Inport  Port=3
  DW1 : Inport  Port=4
  P1W2 : Inport  Port=5
  P3W4 : Inport  Port=6
  OW1 : Inport  Port=7
  OW2 : Inport  Port=8
  OW4 : Inport  Port=9
  LD : Inport  Port=10
  CW1C : Inport  Port=11
  CW2C : Inport  Port=12
  CW4C : Inport  Port=13
  Pri : Subsystem
  Pri3 : Subsystem
  Pri4 : Subsystem
  WL : Subsystem
  WL1 : Subsystem
  WL3 : Subsystem
  W1 : Outport
  W2 : Outport  Port=2
  W4 : Outport  Port=3
  wires:
  CW4C/1 -> Pri4/2(CW4C)
  CW2C/1 -> Pri/2(CW2C)
  CW1C/1 -> Pri3/2(CW1C)
  Pri3/1(User) -> WL/2(User)
  WL3/1(WindowLogicOutput) -> W4/1
  Pri4/1(User) -> WL3/2(User)
  OW4/1 -> WL3/3(OW)
  PosW4/1 -> WL3/1(WPos)
  P3W4/1 -> Pri4/1(P)
  WL1/1(WindowLogicOutput) -> W2/1
  OW2/1 -> WL1/3(OW)
  PosW2/1 -> WL1/1(WPos)
  P1W2/1 -> Pri/1(P)
  Pri/1(User) -> WL1/2(User)
  WL/1(WindowLogicOutput) -> W1/1
  DW1/1 -> Pri3/1(D)
  OW1/1 -> WL/3(OW)
  PosW1/1 -> WL/1(WPos)
  LD/1 -> WL3/4(L)

== system c00019M_harness/M108/Physical ==
  InW1 : Inport
  InW2 : Inport  Port=2
  InW4 : Inport  Port=3
  W : Subsystem
  W5 : Subsystem
  W7 : Subsystem
  W1 : Outport
  W2 : Outport  Port=2
  W4 : Outport  Port=3
  wires:
  W7/1(WPos) -> W4/1
  W5/1(WPos) -> W2/1
  W/1(WPos) -> W1/1
  InW4/1 -> W7/1(WIn)
  InW2/1 -> W5/1(WIn)
  InW1/1 -> W/1(WIn)

== system c00019M_harness/M108/S1 ==
  PhyMeasure : Inport
  SensorOut : Outport
  wires:
  PhyMeasure/1 -> SensorOut/1

== system c00019M_harness/M108/S2 ==
  PhyMeasure : Inport
  SensorOut : Outport
  wires:
  PhyMeasure/1 -> SensorOut/1

== system c00019M_harness/M108/S4 ==
  PhyMeasure : Inport
  SensorOut : Outport
  wires:
  PhyMeasure/1 -> SensorOut/1

== system c00019M_harness/M110/Cyber ==
  note: Sensors
  note: Inputs For Window1
  note: Inputs for Window 2
  note: Inputs for window 3
  note: Inputs for window 4
  note: Users
  note: Users
  note: Sensors
  note: Users
  note: Sensors
  note: Users
  note: Sensors
  note: USERS
      | ---------------------------------
      | 0: None
      | 1: Ventana Arriba
      | 2: Ventana hasta arriba
      | 3: Ventana abajo
      | 4: Ventana hasta abajo
  note: 1: SUBE
      | 0: PARADO
      | -1 BAJA
  note: D = Driver (W1)
      | P1 = Passenger 1 (W2)
      | P2 = Passenger 2 (W3)
      | P3 = Passenger 3 (W4)
      | O = Obstacle
      | C = Control
      | Pri = Prioritizer
      | LD = LockDriver
      | PosW = PositionWindow
      | WL = WindowLogic
      | OW = ObstacleWindow
      | CWXC = ControlWindowXCentralized
      | S = Sensor
      | L = Lock
      | WPos = WindowPosition
      | M = Memory
      | InW = InputWindow
      | WIn = WindowInput
  PosW1 : Inport
  PosW2 : Inport  Port=2
  PosW4 : Inport  Port=3
  DW1 : Inport  Port=4
  P1W2 : Inport  Port=5
  P3W4 : Inport  Port=6
  OW1 : Inport  Port=7
  OW2 : Inport  Port=8
  OW4 : Inport  Port=9
  LD : Inport  Port=10
  CW1C : Inport  Port=11
  CW2C : Inport  Port=12
  CW4C : Inport  Port=13
  Pri : Subsystem
  Pri3 : Subsystem
  Pri4 : Subsystem
  WL : Subsystem
  WL1 : Subsystem
  WL3 : Subsystem
  W1 : Outport
  W2 : Outport  Port=2
  W4 : Outport  Port=3
  wires:
  CW4C/1 -> Pri4/2(CW4C)
  CW2C/1 -> Pri/2(CW2C)
  CW1C/1 -> Pri3/2(CW1C)
  Pri3/1(User) -> WL/2(User)
  WL3/1(WindowLogicOutput) -> W4/1
  Pri4/1(User) -> WL3/2(User)
  OW4/1 -> WL3/3(OW)
  PosW4/1 -> WL3/1(WPos)
  P3W4/1 -> Pri4/1(P)
  WL1/1(WindowLogicOutput) -> W2/1
  OW2/1 -> WL1/3(OW)
  PosW2/1 -> WL1/1(WPos)
  P1W2/1 -> Pri/1(P)
  Pri/1(User) -> WL1/2(User)
  WL/1(WindowLogicOutput) -> W1/1
  DW1/1 -> Pri3/1(D)
  OW1/1 -> WL/3(OW)
  PosW1/1 -> WL/1(WPos)
  LD/1 -> WL3/4(L)

== system c00019M_harness/M110/Physical ==
  InW1 : Inport
  InW2 : Inport  Port=2
  InW4 : Inport  Port=3
  W : Subsystem
  W5 : Subsystem
  W7 : Subsystem
  W1 : Outport
  W2 : Outport  Port=2
  W4 : Outport  Port=3
  wires:
  W7/1(WPos) -> W4/1
  W5/1(WPos) -> W2/1
  W/1(WPos) -> W1/1
  InW4/1 -> W7/1(WIn)
  InW2/1 -> W5/1(WIn)
  InW1/1 -> W/1(WIn)

== system c00019M_harness/M110/S1 ==
  PhyMeasure : Inport
  SensorOut : Outport
  wires:
  PhyMeasure/1 -> SensorOut/1

== system c00019M_harness/M110/S2 ==
  PhyMeasure : Inport
  SensorOut : Outport
  wires:
  PhyMeasure/1 -> SensorOut/1

== system c00019M_harness/M110/S4 ==
  PhyMeasure : Inport
  SensorOut : Outport
  wires:
  PhyMeasure/1 -> SensorOut/1

== system c00019M_harness/M111/Cyber ==
  note: Sensors
  note: Inputs For Window1
  note: Inputs for Window 2
  note: Inputs for window 3
  note: Inputs for window 4
  note: Users
  note: Users
  note: Sensors
  note: Users
  note: Sensors
  note: Users
  note: Sensors
  note: USERS
      | ---------------------------------
      | 0: None
      | 1: Ventana Arriba
      | 2: Ventana hasta arriba
      | 3: Ventana abajo
      | 4: Ventana hasta abajo
  note: 1: SUBE
      | 0: PARADO
      | -1 BAJA
  note: D = Driver (W1)
      | P1 = Passenger 1 (W2)
      | P2 = Passenger 2 (W3)
      | P3 = Passenger 3 (W4)
      | O = Obstacle
      | C = Control
      | Pri = Prioritizer
      | LD = LockDriver
      | PosW = PositionWindow
      | WL = WindowLogic
      | OW = ObstacleWindow
      | CWXC = ControlWindowXCentralized
      | S = Sensor
      | L = Lock
      | WPos = WindowPosition
      | M = Memory
      | InW = InputWindow
      | WIn = WindowInput
  PosW1 : Inport
  PosW2 : Inport  Port=2
  PosW4 : Inport  Port=3
  DW1 : Inport  Port=4
  P1W2 : Inport  Port=5
  P3W4 : Inport  Port=6
  OW1 : Inport  Port=7
  OW2 : Inport  Port=8
  OW4 : Inport  Port=9
  LD : Inport  Port=10
  CW1C : Inport  Port=11
  CW2C : Inport  Port=12
  CW4C : Inport  Port=13
  Pri : Subsystem
  Pri3 : Subsystem
  Pri4 : Subsystem
  WL : Subsystem
  WL1 : Subsystem
  WL3 : Subsystem
  W1 : Outport
  W2 : Outport  Port=2
  W4 : Outport  Port=3
  wires:
  CW4C/1 -> Pri4/2(CW4C)
  CW2C/1 -> Pri/2(CW2C)
  CW1C/1 -> Pri3/2(CW1C)
  Pri3/1(User) -> WL/2(User)
  WL3/1(WindowLogicOutput) -> W4/1
  Pri4/1(User) -> WL3/2(User)
  OW4/1 -> WL3/3(OW)
  PosW4/1 -> WL3/1(WPos)
  P3W4/1 -> Pri4/1(P)
  WL1/1(WindowLogicOutput) -> W2/1
  OW2/1 -> WL1/3(OW)
  PosW2/1 -> WL1/1(WPos)
  P1W2/1 -> Pri/1(P)
  Pri/1(User) -> WL1/2(User)
  WL/1(WindowLogicOutput) -> W1/1
  DW1/1 -> Pri3/1(D)
  OW1/1 -> WL/3(OW)
  PosW1/1 -> WL/1(WPos)
  LD/1 -> WL3/4(L)

== system c00019M_harness/M111/Physical ==
  InW1 : Inport
  InW2 : Inport  Port=2
  InW4 : Inport  Port=3
  W : Subsystem
  W5 : Subsystem
  W7 : Subsystem
  W1 : Outport
  W2 : Outport  Port=2
  W4 : Outport  Port=3
  wires:
  W7/1(WPos) -> W4/1
  W5/1(WPos) -> W2/1
  W/1(WPos) -> W1/1
  InW4/1 -> W7/1(WIn)
  InW2/1 -> W5/1(WIn)
  InW1/1 -> W/1(WIn)

== system c00019M_harness/M111/S1 ==
  PhyMeasure : Inport
  SensorOut : Outport
  wires:
  PhyMeasure/1 -> SensorOut/1

== system c00019M_harness/M111/S2 ==
  PhyMeasure : Inport
  SensorOut : Outport
  wires:
  PhyMeasure/1 -> SensorOut/1

== system c00019M_harness/M111/S4 ==
  PhyMeasure : Inport
  SensorOut : Outport
  wires:
  PhyMeasure/1 -> SensorOut/1

== system c00019M_harness/M112/Cyber ==
  note: Sensors
  note: Inputs For Window1
  note: Inputs for Window 2
  note: Inputs for window 3
  note: Inputs for window 4
  note: Users
  note: Users
  note: Sensors
  note: Users
  note: Sensors
  note: Users
  note: Sensors
  note: USERS
      | ---------------------------------
      | 0: None
      | 1: Ventana Arriba
      | 2: Ventana hasta arriba
      | 3: Ventana abajo
      | 4: Ventana hasta abajo
  note: 1: SUBE
      | 0: PARADO
      | -1 BAJA
  note: D = Driver (W1)
      | P1 = Passenger 1 (W2)
      | P2 = Passenger 2 (W3)
      | P3 = Passenger 3 (W4)
      | O = Obstacle
      | C = Control
      | Pri = Prioritizer
      | LD = LockDriver
      | PosW = PositionWindow
      | WL = WindowLogic
      | OW = ObstacleWindow
      | CWXC = ControlWindowXCentralized
      | S = Sensor
      | L = Lock
      | WPos = WindowPosition
      | M = Memory
      | InW = InputWindow
      | WIn = WindowInput
  PosW1 : Inport
  PosW2 : Inport  Port=2
  PosW4 : Inport  Port=3
  DW1 : Inport  Port=4
  P1W2 : Inport  Port=5
  P3W4 : Inport  Port=6
  OW1 : Inport  Port=7
  OW2 : Inport  Port=8
  OW4 : Inport  Port=9
  LD : Inport  Port=10
  CW1C : Inport  Port=11
  CW2C : Inport  Port=12
  CW4C : Inport  Port=13
  Pri : Subsystem
  Pri3 : Subsystem
  Pri4 : Subsystem
  WL : Subsystem
  WL1 : Subsystem
  WL3 : Subsystem
  W1 : Outport
  W2 : Outport  Port=2
  W4 : Outport  Port=3
  wires:
  CW4C/1 -> Pri4/2(CW4C)
  CW2C/1 -> Pri/2(CW2C)
  CW1C/1 -> Pri3/2(CW1C)
  Pri3/1(User) -> WL/2(User)
  WL3/1(WindowLogicOutput) -> W4/1
  Pri4/1(User) -> WL3/2(User)
  OW4/1 -> WL3/3(OW)
  PosW4/1 -> WL3/1(WPos)
  P3W4/1 -> Pri4/1(P)
  WL1/1(WindowLogicOutput) -> W2/1
  OW2/1 -> WL1/3(OW)
  PosW2/1 -> WL1/1(WPos)
  P1W2/1 -> Pri/1(P)
  Pri/1(User) -> WL1/2(User)
  WL/1(WindowLogicOutput) -> W1/1
  DW1/1 -> Pri3/1(D)
  OW1/1 -> WL/3(OW)
  PosW1/1 -> WL/1(WPos)
  LD/1 -> WL3/4(L)

== system c00019M_harness/M112/Physical ==
  InW1 : Inport
  InW2 : Inport  Port=2
  InW4 : Inport  Port=3
  W : Subsystem
  W5 : Subsystem
  W7 : Subsystem
  W1 : Outport
  W2 : Outport  Port=2
  W4 : Outport  Port=3
  wires:
  W7/1(WPos) -> W4/1
  W5/1(WPos) -> W2/1
  W/1(WPos) -> W1/1
  InW4/1 -> W7/1(WIn)
  InW2/1 -> W5/1(WIn)
  InW1/1 -> W/1(WIn)

== system c00019M_harness/M112/S1 ==
  PhyMeasure : Inport
  SensorOut : Outport
  wires:
  PhyMeasure/1 -> SensorOut/1

== system c00019M_harness/M112/S2 ==
  PhyMeasure : Inport
  SensorOut : Outport
  wires:
  PhyMeasure/1 -> SensorOut/1

== system c00019M_harness/M112/S4 ==
  PhyMeasure : Inport
  SensorOut : Outport
  wires:
  PhyMeasure/1 -> SensorOut/1

== system c00019M_harness/M114/Cyber ==
  note: Sensors
  note: Inputs For Window1
  note: Inputs for Window 2
  note: Inputs for window 3
  note: Inputs for window 4
  note: Users
  note: Users
  note: Sensors
  note: Users
  note: Sensors
  note: Users
  note: Sensors
  note: USERS
      | ---------------------------------
      | 0: None
      | 1: Ventana Arriba
      | 2: Ventana hasta arriba
      | 3: Ventana abajo
      | 4: Ventana hasta abajo
  note: 1: SUBE
      | 0: PARADO
      | -1 BAJA
  note: D = Driver (W1)
      | P1 = Passenger 1 (W2)
      | P2 = Passenger 2 (W3)
      | P3 = Passenger 3 (W4)
      | O = Obstacle
      | C = Control
      | Pri = Prioritizer
      | LD = LockDriver
      | PosW = PositionWindow
      | WL = WindowLogic
      | OW = ObstacleWindow
      | CWXC = ControlWindowXCentralized
      | S = Sensor
      | L = Lock
      | WPos = WindowPosition
      | M = Memory
      | InW = InputWindow
      | WIn = WindowInput
  PosW1 : Inport
  PosW2 : Inport  Port=2
  PosW4 : Inport  Port=3
  DW1 : Inport  Port=4
  P1W2 : Inport  Port=5
  P3W4 : Inport  Port=6
  OW1 : Inport  Port=7
  OW2 : Inport  Port=8
  OW4 : Inport  Port=9
  LD : Inport  Port=10
  CW1C : Inport  Port=11
  CW2C : Inport  Port=12
  CW4C : Inport  Port=13
  Pri : Subsystem
  Pri3 : Subsystem
  Pri4 : Subsystem
  WL : Subsystem
  WL1 : Subsystem
  WL3 : Subsystem
  W1 : Outport
  W2 : Outport  Port=2
  W4 : Outport  Port=3
  wires:
  CW4C/1 -> Pri4/2(CW4C)
  CW2C/1 -> Pri/2(CW2C)
  CW1C/1 -> Pri3/2(CW1C)
  Pri3/1(User) -> WL/2(User)
  WL3/1(WindowLogicOutput) -> W4/1
  Pri4/1(User) -> WL3/2(User)
  OW4/1 -> WL3/3(OW)
  PosW4/1 -> WL3/1(WPos)
  P3W4/1 -> Pri4/1(P)
  WL1/1(WindowLogicOutput) -> W2/1
  OW2/1 -> WL1/3(OW)
  PosW2/1 -> WL1/1(WPos)
  P1W2/1 -> Pri/1(P)
  Pri/1(User) -> WL1/2(User)
  WL/1(WindowLogicOutput) -> W1/1
  DW1/1 -> Pri3/1(D)
  OW1/1 -> WL/3(OW)
  PosW1/1 -> WL/1(WPos)
  LD/1 -> WL3/4(L)

== system c00019M_harness/M114/Physical ==
  InW1 : Inport
  InW2 : Inport  Port=2
  InW4 : Inport  Port=3
  W : Subsystem
  W5 : Subsystem
  W7 : Subsystem
  W1 : Outport
  W2 : Outport  Port=2
  W4 : Outport  Port=3
  wires:
  W7/1(WPos) -> W4/1
  W5/1(WPos) -> W2/1
  W/1(WPos) -> W1/1
  InW4/1 -> W7/1(WIn)
  InW2/1 -> W5/1(WIn)
  InW1/1 -> W/1(WIn)

== system c00019M_harness/M114/S1 ==
  PhyMeasure : Inport
  SensorOut : Outport
  wires:
  PhyMeasure/1 -> SensorOut/1

== system c00019M_harness/M114/S2 ==
  PhyMeasure : Inport
  SensorOut : Outport
  wires:
  PhyMeasure/1 -> SensorOut/1

== system c00019M_harness/M114/S4 ==
  PhyMeasure : Inport
  SensorOut : Outport
  wires:
  PhyMeasure/1 -> SensorOut/1

== system c00019M_harness/M115/Cyber ==
  note: Sensors
  note: Inputs For Window1
  note: Inputs for Window 2
  note: Inputs for window 3
  note: Inputs for window 4
  note: Users
  note: Users
  note: Sensors
  note: Users
  note: Sensors
  note: Users
  note: Sensors
  note: USERS
      | ---------------------------------
      | 0: None
      | 1: Ventana Arriba
      | 2: Ventana hasta arriba
      | 3: Ventana abajo
      | 4: Ventana hasta abajo
  note: 1: SUBE
      | 0: PARADO
      | -1 BAJA
  note: D = Driver (W1)
      | P1 = Passenger 1 (W2)
      | P2 = Passenger 2 (W3)
      | P3 = Passenger 3 (W4)
      | O = Obstacle
      | C = Control
      | Pri = Prioritizer
      | LD = LockDriver
      | PosW = PositionWindow
      | WL = WindowLogic
      | OW = ObstacleWindow
      | CWXC = ControlWindowXCentralized
      | S = Sensor
      | L = Lock
      | WPos = WindowPosition
      | M = Memory
      | InW = InputWindow
      | WIn = WindowInput
  PosW1 : Inport
  PosW2 : Inport  Port=2
  PosW4 : Inport  Port=3
  DW1 : Inport  Port=4
  P1W2 : Inport  Port=5
  P3W4 : Inport  Port=6
  OW1 : Inport  Port=7
  OW2 : Inport  Port=8
  OW4 : Inport  Port=9
  LD : Inport  Port=10
  CW1C : Inport  Port=11
  CW2C : Inport  Port=12
  CW4C : Inport  Port=13
  Pri : Subsystem
  Pri3 : Subsystem
  Pri4 : Subsystem
  WL : Subsystem
  WL1 : Subsystem
  WL3 : Subsystem
  W1 : Outport
  W2 : Outport  Port=2
  W4 : Outport  Port=3
  wires:
  CW4C/1 -> Pri4/2(CW4C)
  CW2C/1 -> Pri/2(CW2C)
  CW1C/1 -> Pri3/2(CW1C)
  Pri3/1(User) -> WL/2(User)
  WL3/1(WindowLogicOutput) -> W4/1
  Pri4/1(User) -> WL3/2(User)
  OW4/1 -> WL3/3(OW)
  PosW4/1 -> WL3/1(WPos)
  P3W4/1 -> Pri4/1(P)
  WL1/1(WindowLogicOutput) -> W2/1
  OW2/1 -> WL1/3(OW)
  PosW2/1 -> WL1/1(WPos)
  P1W2/1 -> Pri/1(P)
  Pri/1(User) -> WL1/2(User)
  WL/1(WindowLogicOutput) -> W1/1
  DW1/1 -> Pri3/1(D)
  OW1/1 -> WL/3(OW)
  PosW1/1 -> WL/1(WPos)
  LD/1 -> WL3/4(L)

== system c00019M_harness/M115/Physical ==
  InW1 : Inport
  InW2 : Inport  Port=2
  InW4 : Inport  Port=3
  W : Subsystem
  W5 : Subsystem
  W7 : Subsystem
  W1 : Outport
  W2 : Outport  Port=2
  W4 : Outport  Port=3
  wires:
  W7/1(WPos) -> W4/1
  W5/1(WPos) -> W2/1
  W/1(WPos) -> W1/1
  InW4/1 -> W7/1(WIn)
  InW2/1 -> W5/1(WIn)
  InW1/1 -> W/1(WIn)

== system c00019M_harness/M115/S1 ==
  PhyMeasure : Inport
  SensorOut : Outport
  wires:
  PhyMeasure/1 -> SensorOut/1

== system c00019M_harness/M115/S2 ==
  PhyMeasure : Inport
  SensorOut : Outport
  wires:
  PhyMeasure/1 -> SensorOut/1

== system c00019M_harness/M115/S4 ==
  PhyMeasure : Inport
  SensorOut : Outport
  wires:
  PhyMeasure/1 -> SensorOut/1

== system c00019M_harness/M116/Cyber ==
  note: Sensors
  note: Inputs For Window1
  note: Inputs for Window 2
  note: Inputs for window 3
  note: Inputs for window 4
  note: Users
  note: Users
  note: Sensors
  note: Users
  note: Sensors
  note: Users
  note: Sensors
  note: USERS
      | ---------------------------------
      | 0: None
      | 1: Ventana Arriba
      | 2: Ventana hasta arriba
      | 3: Ventana abajo
      | 4: Ventana hasta abajo
  note: 1: SUBE
      | 0: PARADO
      | -1 BAJA
  note: D = Driver (W1)
      | P1 = Passenger 1 (W2)
      | P2 = Passenger 2 (W3)
      | P3 = Passenger 3 (W4)
      | O = Obstacle
      | C = Control
      | Pri = Prioritizer
      | LD = LockDriver
      | PosW = PositionWindow
      | WL = WindowLogic
      | OW = ObstacleWindow
      | CWXC = ControlWindowXCentralized
      | S = Sensor
      | L = Lock
      | WPos = WindowPosition
      | M = Memory
      | InW = InputWindow
      | WIn = WindowInput
  PosW1 : Inport
  PosW2 : Inport  Port=2
  PosW4 : Inport  Port=3
  DW1 : Inport  Port=4
  P1W2 : Inport  Port=5
  P3W4 : Inport  Port=6
  OW1 : Inport  Port=7
  OW2 : Inport  Port=8
  OW4 : Inport  Port=9
  LD : Inport  Port=10
  CW1C : Inport  Port=11
  CW2C : Inport  Port=12
  CW4C : Inport  Port=13
  Pri : Subsystem
  Pri3 : Subsystem
  Pri4 : Subsystem
  WL : Subsystem
  WL1 : Subsystem
  WL3 : Subsystem
  W1 : Outport
  W2 : Outport  Port=2
  W4 : Outport  Port=3
  wires:
  CW4C/1 -> Pri4/2(CW4C)
  CW2C/1 -> Pri/2(CW2C)
  CW1C/1 -> Pri3/2(CW1C)
  Pri3/1(User) -> WL/2(User)
  WL3/1(WindowLogicOutput) -> W4/1
  Pri4/1(User) -> WL3/2(User)
  OW4/1 -> WL3/3(OW)
  PosW4/1 -> WL3/1(WPos)
  P3W4/1 -> Pri4/1(P)
  WL1/1(WindowLogicOutput) -> W2/1
  OW2/1 -> WL1/3(OW)
  PosW2/1 -> WL1/1(WPos)
  P1W2/1 -> Pri/1(P)
  Pri/1(User) -> WL1/2(User)
  WL/1(WindowLogicOutput) -> W1/1
  DW1/1 -> Pri3/1(D)
  OW1/1 -> WL/3(OW)
  PosW1/1 -> WL/1(WPos)
  LD/1 -> WL3/4(L)

== system c00019M_harness/M116/Physical ==
  InW1 : Inport
  InW2 : Inport  Port=2
  InW4 : Inport  Port=3
  W : Subsystem
  W5 : Subsystem
  W7 : Subsystem
  W1 : Outport
  W2 : Outport  Port=2
  W4 : Outport  Port=3
  wires:
  W7/1(WPos) -> W4/1
  W5/1(WPos) -> W2/1
  W/1(WPos) -> W1/1
  InW4/1 -> W7/1(WIn)
  InW2/1 -> W5/1(WIn)
  InW1/1 -> W/1(WIn)

== system c00019M_harness/M116/S1 ==
  PhyMeasure : Inport
  SensorOut : Outport
  wires:
  PhyMeasure/1 -> SensorOut/1

== system c00019M_harness/M116/S2 ==
  PhyMeasure : Inport
  SensorOut : Outport
  wires:
  PhyMeasure/1 -> SensorOut/1

== system c00019M_harness/M116/S4 ==
  PhyMeasure : Inport
  SensorOut : Outport
  wires:
  PhyMeasure/1 -> SensorOut/1

== system c00019M_harness/M118/Cyber ==
  note: Sensors
  note: Inputs For Window1
  note: Inputs for Window 2
  note: Inputs for window 3
  note: Inputs for window 4
  note: Users
  note: Users
  note: Sensors
  note: Users
  note: Sensors
  note: Users
  note: Sensors
  note: USERS
      | ---------------------------------
      | 0: None
      | 1: Ventana Arriba
      | 2: Ventana hasta arriba
      | 3: Ventana abajo
      | 4: Ventana hasta abajo
  note: 1: SUBE
      | 0: PARADO
      | -1 BAJA
  note: D = Driver (W1)
      | P1 = Passenger 1 (W2)
      | P2 = Passenger 2 (W3)
      | P3 = Passenger 3 (W4)
      | O = Obstacle
      | C = Control
      | Pri = Prioritizer
      | LD = LockDriver
      | PosW = PositionWindow
      | WL = WindowLogic
      | OW = ObstacleWindow
      | CWXC = ControlWindowXCentralized
      | S = Sensor
      | L = Lock
      | WPos = WindowPosition
      | M = Memory
      | InW = InputWindow
      | WIn = WindowInput
  PosW1 : Inport
  PosW2 : Inport  Port=2
  PosW4 : Inport  Port=3
  DW1 : Inport  Port=4
  P1W2 : Inport  Port=5
  P3W4 : Inport  Port=6
  OW1 : Inport  Port=7
  OW2 : Inport  Port=8
  OW4 : Inport  Port=9
  LD : Inport  Port=10
  CW1C : Inport  Port=11
  CW2C : Inport  Port=12
  CW4C : Inport  Port=13
  Pri : Subsystem
  Pri3 : Subsystem
  Pri4 : Subsystem
  WL : Subsystem
  WL1 : Subsystem
  WL3 : Subsystem
  W1 : Outport
  W2 : Outport  Port=2
  W4 : Outport  Port=3
  wires:
  CW4C/1 -> Pri4/2(CW4C)
  CW2C/1 -> Pri/2(CW2C)
  CW1C/1 -> Pri3/2(CW1C)
  Pri3/1(User) -> WL/2(User)
  WL3/1(WindowLogicOutput) -> W4/1
  Pri4/1(User) -> WL3/2(User)
  OW4/1 -> WL3/3(OW)
  PosW4/1 -> WL3/1(WPos)
  P3W4/1 -> Pri4/1(P)
  WL1/1(WindowLogicOutput) -> W2/1
  OW2/1 -> WL1/3(OW)
  PosW2/1 -> WL1/1(WPos)
  P1W2/1 -> Pri/1(P)
  Pri/1(User) -> WL1/2(User)
  WL/1(WindowLogicOutput) -> W1/1
  DW1/1 -> Pri3/1(D)
  OW1/1 -> WL/3(OW)
  PosW1/1 -> WL/1(WPos)
  LD/1 -> WL3/4(L)

== system c00019M_harness/M118/Physical ==
  InW1 : Inport
  InW2 : Inport  Port=2
  InW4 : Inport  Port=3
  W : Subsystem
  W5 : Subsystem
  W7 : Subsystem
  W1 : Outport
  W2 : Outport  Port=2
  W4 : Outport  Port=3
  wires:
  W7/1(WPos) -> W4/1
  W5/1(WPos) -> W2/1
  W/1(WPos) -> W1/1
  InW4/1 -> W7/1(WIn)
  InW2/1 -> W5/1(WIn)
  InW1/1 -> W/1(WIn)

== system c00019M_harness/M118/S1 ==
  PhyMeasure : Inport
  SensorOut : Outport
  wires:
  PhyMeasure/1 -> SensorOut/1

== system c00019M_harness/M118/S2 ==
  PhyMeasure : Inport
  SensorOut : Outport
  wires:
  PhyMeasure/1 -> SensorOut/1

== system c00019M_harness/M118/S4 ==
  PhyMeasure : Inport
  SensorOut : Outport
  wires:
  PhyMeasure/1 -> SensorOut/1

== system c00019M_harness/M119/Cyber ==
  note: Sensors
  note: Inputs For Window1
  note: Inputs for Window 2
  note: Inputs for window 3
  note: Inputs for window 4
  note: Users
  note: Users
  note: Sensors
  note: Users
  note: Sensors
  note: Users
  note: Sensors
  note: USERS
      | ---------------------------------
      | 0: None
      | 1: Ventana Arriba
      | 2: Ventana hasta arriba
      | 3: Ventana abajo
      | 4: Ventana hasta abajo
  note: 1: SUBE
      | 0: PARADO
      | -1 BAJA
  note: D = Driver (W1)
      | P1 = Passenger 1 (W2)
      | P2 = Passenger 2 (W3)
      | P3 = Passenger 3 (W4)
      | O = Obstacle
      | C = Control
      | Pri = Prioritizer
      | LD = LockDriver
      | PosW = PositionWindow
      | WL = WindowLogic
      | OW = ObstacleWindow
      | CWXC = ControlWindowXCentralized
      | S = Sensor
      | L = Lock
      | WPos = WindowPosition
      | M = Memory
      | InW = InputWindow
      | WIn = WindowInput
  PosW1 : Inport
  PosW2 : Inport  Port=2
  PosW4 : Inport  Port=3
  DW1 : Inport  Port=4
  P1W2 : Inport  Port=5
  P3W4 : Inport  Port=6
  OW1 : Inport  Port=7
  OW2 : Inport  Port=8
  OW4 : Inport  Port=9
  LD : Inport  Port=10
  CW1C : Inport  Port=11
  CW2C : Inport  Port=12
  CW4C : Inport  Port=13
  Pri : Subsystem
  Pri3 : Subsystem
  Pri4 : Subsystem
  WL : Subsystem
  WL1 : Subsystem
  WL3 : Subsystem
  W1 : Outport
  W2 : Outport  Port=2
  W4 : Outport  Port=3
  wires:
  CW4C/1 -> Pri4/2(CW4C)
  CW2C/1 -> Pri/2(CW2C)
  CW1C/1 -> Pri3/2(CW1C)
  Pri3/1(User) -> WL/2(User)
  WL3/1(WindowLogicOutput) -> W4/1
  Pri4/1(User) -> WL3/2(User)
  OW4/1 -> WL3/3(OW)
  PosW4/1 -> WL3/1(WPos)
  P3W4/1 -> Pri4/1(P)
  WL1/1(WindowLogicOutput) -> W2/1
  OW2/1 -> WL1/3(OW)
  PosW2/1 -> WL1/1(WPos)
  P1W2/1 -> Pri/1(P)
  Pri/1(User) -> WL1/2(User)
  WL/1(WindowLogicOutput) -> W1/1
  DW1/1 -> Pri3/1(D)
  OW1/1 -> WL/3(OW)
  PosW1/1 -> WL/1(WPos)
  LD/1 -> WL3/4(L)

== system c00019M_harness/M119/Physical ==
  InW1 : Inport
  InW2 : Inport  Port=2
  InW4 : Inport  Port=3
  W : Subsystem
  W5 : Subsystem
  W7 : Subsystem
  W1 : Outport
  W2 : Outport  Port=2
  W4 : Outport  Port=3
  wires:
  W7/1(WPos) -> W4/1
  W5/1(WPos) -> W2/1
  W/1(WPos) -> W1/1
  InW4/1 -> W7/1(WIn)
  InW2/1 -> W5/1(WIn)
  InW1/1 -> W/1(WIn)

== system c00019M_harness/M119/S1 ==
  PhyMeasure : Inport
  SensorOut : Outport
  wires:
  PhyMeasure/1 -> SensorOut/1

== system c00019M_harness/M119/S2 ==
  PhyMeasure : Inport
  SensorOut : Outport
  wires:
  PhyMeasure/1 -> SensorOut/1

== system c00019M_harness/M119/S4 ==
  PhyMeasure : Inport
  SensorOut : Outport
  wires:
  PhyMeasure/1 -> SensorOut/1
